simulink model "FW_Matlab_main"  (R2024b)
settings: Solver=ode4  StartTime=0.0  StopTime=inf  FixedStep=0.001  RelTol=1e-3
model workspace (MAT data in the model file):
  freq = 1
libraries: eeGeneralControl x8, slrealtimeiplib x5, cstblocks x3, simulink_extras x2, vrlib x1, aerolibanimutils x1, dspnetwork x1
(part 1 of 2)
settings Model: Creator=s336079  LastModifiedBy=user
settings SolverCC: AlgebraicLoopSolver=TrustRegion
settings DebuggingCC: UnconnectedInputMsg=warning  UnconnectedOutputMsg=warning  UnconnectedLineMsg=warning
settings ModelReferenceCC: EnableRefExpFcnMdlSchedulingChecks=on
settings RTWCC: GPUComputeCapability=3.5

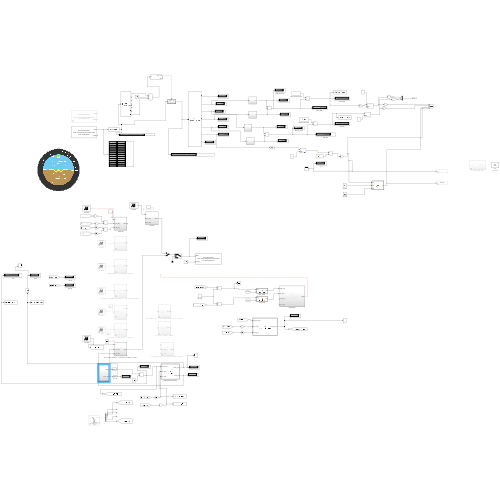
[thumbnail: Simulink's stored preview of the top-level diagram]
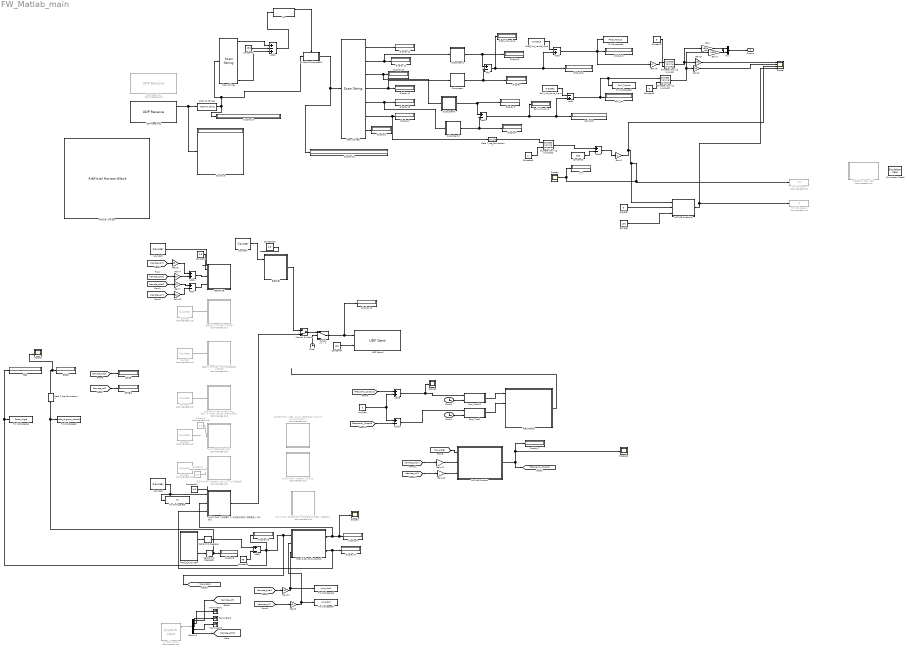
== system FW_Matlab_main ==
  10.27 想做对称推力测试 : Subsystem  Commented=on
  ASCII to String2 : ASCIIToString
  Add{,2,5,7..8,10} (6 alike) : Sum  Inputs=+-
  Add1 : Sum  Inputs=+-+
  Add3 : Sum  Inputs=-+
  Add4 : Sum  Inputs=-+
  Add6 : Sum
  Add9 : Sum
  Artificial Horizon : ArtificialHorizonBlock
  Clock : Clock
  Clock1 : Clock
  Clock2 : Clock
  Constant : Constant  Value=0.8
  Constant1 : Constant  Value=130
  Constant10 : Constant  Value=0.8
  Constant11 : Constant  Value=0.8
  Constant2 : Constant  Commented=on  Value=0.8
  Constant3 : Constant  Value=433
  Constant4 : Constant  Value=100
  Constant5 : Constant  Value=98
  Constant6 : Constant  Commented=on  Value=0.8
  Constant7 : Constant  Value=5
  Constant8 : Constant  Value=5
  Constant9 : Constant  Value=2
  Counter : eeGeneralControl/Counter  Commented=on  CarrCount=Up  Range=[0 1]  Tper=1/5  Tdelay=0  Ts=0.001
  Counter1 : eeGeneralControl/Counter  Commented=on  CarrCount=Up  Range=[0 1]  Tper=1/5  Tdelay=0  Ts=0.001
  Counter2 : eeGeneralControl/Counter  Commented=on  CarrCount=Up  Range=[0 1]  Tper=1/1  Tdelay=0  Ts=0.001
  Counter3 : eeGeneralControl/Counter  Commented=on  CarrCount=Up  Range=[0 1]  Tper=3  Tdelay=0  Ts=0.001
  Counter4 : eeGeneralControl/Counter  Commented=on  CarrCount=Up  Range=[0 1]  Tper=1/5  Tdelay=0  Ts=0.001
  Counter5 : eeGeneralControl/Counter  CarrCount=Up  Range=[0 1]  Tper=1/1  Tdelay=0  Ts=0.001
  Counter6 : eeGeneralControl/Counter  CarrCount=Up  Range=[0 1]  Tper=1/0.1  Tdelay=0  Ts=0.001
  Counter7 : eeGeneralControl/Counter  CarrCount=Up  Range=[0 1]  Tper=1/3  Tdelay=0  Ts=0.001
  Data Type Conversion1 : DataTypeConversion  OutDataTypeStr=double  SaturateOnIntegerOverflow=off  RndMeth=Floor
  Data Type Conversion4 : DataTypeConversion  OutDataTypeStr=double  SaturateOnIntegerOverflow=off  RndMeth=Floor
  Demux1 : Demux  Outputs=5
  Discrete Varying Lowpass : cstblocks/Linear Parameter Varying/Discrete Varying Lowpass  N=1  w0=0  Ts=0.001
  Discrete Varying Lowpass1 : cstblocks/Linear Parameter Varying/Discrete Varying Lowpass  N=1  w0=0  Ts=0.001
  Discrete Varying Lowpass2 : cstblocks/Linear Parameter Varying/Discrete Varying Lowpass  N=1  w0=0  Ts=0.001
  Display{,1..19} (20 alike) : Display
  FWR_Z_AXIS UDP : Subsystem
  Gain : Gain  Gain=1500
  Gain1 : Gain  Gain=1500
  Gain10 : Gain  Gain=20
  Gain11 : Gain  Gain=40
  Gain12 : Gain  Gain=0.01
  Gain13 : Gain  Gain=0.01
  Gain2 : Gain  Gain=-1
  Gain3 : Gain  Gain=40
  Gain4 : Gain  Gain=50
  Gain5 : Gain  Gain=200
  Gain6 : Gain  Gain=200
  Gain7 : Gain  Gain=50
  Gain8 : Gain  Gain=-1
  Gain9 : Gain  Gain=20
  If Action Subsystem2 : Subsystem  TreatAsAtomicUnit=on
  If2 : If  IfExpression=u1 == 0
  Init_Freq : Constant  Value=5
  Joystick Input1 : vrlib/Joystick Input  Commented=on  joyid=1  adjustports=on  forcefeed=off
  MATLAB Function : MATLAB Function  TreatAsAtomicUnit=on
  MATLAB Function6 : MATLAB Function  TreatAsAtomicUnit=on
  Manual Switch1 : ManualSwitch  CurrentSetting=0
  Msc 期间升力最大FWR模式 Msc 期间工作（拍幅：50/-20 扭转角10/50） : Subsystem  Commented=on
  Mux : Mux  Inputs=2
  Pitch_NM : Display
  Pitch_NM1 : Display
  Pitch_init_valve : Display
  Pitch_init_valve_input : Constant  Value=-0.01018
  Radians to Degrees : simulink_extras/Transformations/Radians to Degrees
  Radians to Degrees1 : simulink_extras/Transformations/Radians to Degrees
  Roll_NM : Display
  Roll_NM1 : Display
  Roll_init_valve : Display
  Roll_init_valve_input : Constant  Value=-0.02692
  Saw_Tooth : MATLAB Function  TreatAsAtomicUnit=on
  Saw_Tooth1 : MATLAB Function  TreatAsAtomicUnit=on
  Scan String3 : ScanString  Format="\"%f\\t%f\\t%f\\t%f\\t%f\\t%f\\t%f\\t\""
  Scan String4 : ScanString  Format="\"%f\\t%f\\t%f\\t%f\\t%f\\t%f\\t%f\\t\""
  Scope : Scope  NumInputPorts=4
  Scope1 : Scope  NumInputPorts=2
  Scope{2..4,10} (4 alike) : Scope
  Simulation Pace1 : aerolibanimutils/Simulation Pace  SimulationPace=1  SleepMode=Auto  OutputPaceError=off  SampleTime=0.001
  Subsystem : Subsystem
  Subsystem1 : Subsystem
  Subsystem2 : Subsystem
  Subsystem3 : Subsystem
  Switch : Switch  Criteria=u2 > Threshold  Threshold=5  SaturateOnIntegerOverflow=off  InputSameDT=off
  Terminator1 : Terminator
  Terminator2 : Terminator
  Terminator3 : Terminator
  To Workspace : ToWorkspace  Commented=on  VariableName=Lift  SaveFormat=Timeseries  SampleTime=-1
  To Workspace1 : ToWorkspace  Commented=on  VariableName=Cl  SaveFormat=Timeseries  SampleTime=-1
  To Workspace2 : ToWorkspace  VariableName=Rotor_Angle  SaveFormat=Timeseries  SampleTime=-1
  To Workspace3 : ToWorkspace  VariableName=Rotor_Angular_Velocity  SaveFormat=Timeseries  SampleTime=-1
  To Workspace4 : ToWorkspace  VariableName=Pitch_Torque  SaveFormat=Timeseries  SampleTime=-1
  To Workspace5 : ToWorkspace  VariableName=Roll_Torque  SaveFormat=Timeseries  SampleTime=-1
  To Workspace6 : ToWorkspace  VariableName=Amp_Pitch  SaveFormat=Timeseries  SampleTime=-1
  To Workspace7 : ToWorkspace  VariableName=Amp_Roll  SaveFormat=Timeseries  SampleTime=-1
  To Workspace8 : ToWorkspace  VariableName=Hz  SaveFormat=Timeseries  SampleTime=-1
  Total Pitch Cyclic Control : MATLAB Function  TreatAsAtomicUnit=on
  UDP Receive1 : slrealtimeiplib/UDP Receive  Commented=on  useHostTargetConn=on  ipAddress=10.10.10.15  localPort=2315  rcvWidth=1024  rcvFmAny=off  fmAddress=192.168.0.30  sampleTime=-1  enableMessage=off  maxPackets=1
  UDP Receive2 : slrealtimeiplib/UDP Receive  useHostTargetConn=on  ipAddress=10.10.10.15  localPort=2318  rcvWidth=1024  rcvFmAny=on  fmAddress=192.168.0.51  sampleTime=-1  enableMessage=off  maxPackets=1
  UDP Send1 : slrealtimeiplib/UDP Send  useHostTargetConn=on  toAddress=192.168.0.52  toPort=2316  sampleTime=-1  enableMessage=off  localPort=25001
  两翼分频控制 : Subsystem
  优化中 FWR- 尝试姿态控制-小拍动幅度-新小幅度（周期变距） : Subsystem  Commented=on
  优化中 FWR（当前最优）- 尝试姿态控制（周期变距）124 测王 : Subsystem
  优化中 FWR（当前最优）10.29前 : Subsystem  Commented=on
  优化中 FWR（当前最优）10.29后，改了扭转角度 : Subsystem  Commented=on
  升力 : Display
  "启动测力台 UDP  接收 " : Subsystem  Commented=on
  拍动频率 : Constant  Value=5
  推杆量 : Display
  推杆量1 : Display
  普通扑翼 : Subsystem
  最大拍幅 : Constant  Value=120
  蜻蜓扑动-FWR模式-角度与普通蜻蜓同  45度范围 : Subsystem  Commented=on
  蜻蜓扑动-VTOL模式 45度范围 : Subsystem  Commented=on
  蜻蜓改扑翼 : Subsystem
  角度 : Display
  角速度 : Display
  论文模式 FWR（拍幅：10/-10 扭转角5/25）Cl5.11? 升力没论文说的大 1 : Subsystem  Commented=on
  Output : Outport
  wires:
  Scan String4/1 -> Add1/1
  Scan String3/5 -> Subsystem2/1(In1), Display15/1
  Scan String3/1 -> Display11/1
  Scan String4/7 -> Add1/3
  If2/1 -> If Action Subsystem2/Action
  Scan String3/2 -> Subsystem1/1(In1), Display12/1
  Constant1/1 -> Add1/2
  ASCII to String2/1 -> If Action Subsystem2/1(In1), Scan String4/1, Display10/1
  Add1/1 -> If2/1
  Scan String3/4 -> Subsystem/1(In1), Display14/1
  UDP Receive2/1 -> Display6/1, ASCII to String2/1
  If Action Subsystem2/1(Out1) -> Display16/1, Scan String3/1
  Scan String3/6 -> Data Type Conversion1/1, Display2/1
  Scan String3/3 -> Subsystem3/1(In1), Display13/1
  Scan String3/7 -> Display1/1
  Subsystem/1(Out1) -> Add/2, Display/1
  Subsystem1/1(Out1) -> Add/1, Display3/1
  Add/1 -> Add3/2, Pitch_NM1/1, Pitch_init_valve/1
  Subsystem3/1(Out1) -> Display5/1, Add2/1
  Subsystem2/1(Out1) -> Add2/2, Display4/1
  Pitch_init_valve_input/1 -> Add3/1
  Add3/1 -> To Workspace4/1, Gain8/1, Pitch_NM/1
  Roll_init_valve_input/1 -> Add4/1
  Add4/1 -> To Workspace5/1, Discrete Varying Lowpass1/1, Roll_NM/1
  Add2/1 -> Roll_init_valve/1, Add4/2, Roll_NM1/1
  Mux/1 -> Output/1
  Gain/1 -> Mux/2
  Gain1/1 -> Mux/1
  Constant3/1 -> Add5/2
  Add5/1 -> Gain2/1
  Gain5/1 -> Scope/1
  Gain6/1 -> Scope/2
  Demux1/3 -> Terminator2/1
  Demux1/2 -> Terminator1/1
  Demux1/4 -> Terminator3/1
  Demux1/5 -> [remote_pitch]
  Demux1/1 -> [remote_roll]
  Joystick Input1/1 -> Demux1/1
  拍动频率/1 -> MATLAB Function6/2(freq)
  最大拍幅/1 -> MATLAB Function6/3(Amp)
  MATLAB Function6/1(Cl) -> Scope/4, To Workspace1/1
  Counter/1 -> 蜻蜓扑动-VTOL模式 45度范围/1(In1)
  Counter1/1 -> 蜻蜓扑动-FWR模式-角度与普通蜻蜓同  45度范围/1(In1)
  Constant4/1 -> UDP Send1/2
  Switch/1 -> Display19/1, UDP Send1/1
  Counter2/1 -> Msc 期间升力最大FWR模式 Msc 期间工作（拍幅：50/-20 扭转角10/50）/1(In1)
  Clock/1 -> Switch/2
  Manual Switch1/1 -> Switch/1
  Counter3/1 -> ?
  优化中 FWR（当前最优）- 尝试姿态控制（周期变距）124 测王/1(Signal) -> Manual Switch1/2
  Counter4/1 -> 优化中 FWR（当前最优）10.29后，改了扭转角度/1(In1)
  Counter5/1 -> ?
  普通扑翼/1(Signal) -> Manual Switch1/1
  FWR_Z_AXIS UDP/1(Angle) -> Radians to Degrees/1
  Counter6/1 -> 优化中 FWR（当前最优）- 尝试姿态控制（周期变距）124 测王/1(In1), To Workspace8/1
  Total Pitch Cyclic Control/1(blade_right) -> 优化中 FWR（当前最优）- 尝试姿态控制（周期变距）124 测王/2(R_Pit_Ang), Scope2/1, Display9/1
  Total Pitch Cyclic Control/2(blade_left) -> 优化中 FWR（当前最优）- 尝试姿态控制（周期变距）124 测王/3(L_Pit_Ang), Display17/1
  Constant2/1 -> ?
  Data Type Conversion4/1 -> Scope1/2, 角速度/1
  [remote_pitch] -> Gain4/1
  Gain4/1 -> Add6/2
  [remote_pitch] -> Gain7/1
  Gain7/1 -> Add7/1
  Constant/1 -> 蜻蜓改扑翼/1(In1)
  Gain8/1 -> Discrete Varying Lowpass/1
  Add6/1 -> 蜻蜓改扑翼/2(R_Pit_Ang)
  [remote_roll] -> Gain9/1
  [remote_roll] -> Gain10/1
  Add7/1 -> 蜻蜓改扑翼/3(L_Pit_Ang)
  Gain9/1 -> Add6/1
  Gain10/1 -> Add7/2
  FWR_Z_AXIS UDP/2(Angle_Vel) -> Radians to Degrees1/1
  Radians to Degrees/1 -> Add8/1
  Radians to Degrees1/1 -> To Workspace3/1, Data Type Conversion4/1, Display8/1
  Constant5/1 -> Add8/2
  [remote_pitch] -> Gain11/1
  Gain3/1 -> To Workspace7/1, Total Pitch Cyclic Control/2(Amp_Roll)
  [remote_pitch] -> 推杆量/1
  [remote_roll] -> Gain3/1
  Discrete Varying Lowpass/1 -> Gain/1, Gain5/1
  Discrete Varying Lowpass1/1 -> Gain1/1, Gain6/1
  Constant7/1 -> Discrete Varying Lowpass/2
  Constant8/1 -> Discrete Varying Lowpass1/2
  Gain11/1 -> To Workspace6/1, Total Pitch Cyclic Control/3(Amp_Pitch)
  [remote_roll] -> 推杆量1/1
  Discrete Varying Lowpass2/1 -> Add5/1
  Constant9/1 -> Discrete Varying Lowpass2/2
  Data Type Conversion1/1 -> Discrete Varying Lowpass2/1
  Counter7/1 -> 普通扑翼/1(In1)
  两翼分频控制/1(Signal) -> ?
  [Az_Angle] -> MATLAB Function/1(Azimuth_Angle)
  MATLAB Function/1(Freq_diff_out) -> [Frequency_Output], Scope10/1, Display7/1
  Clock1/1 -> Saw_Tooth/2(t)
  Add10/1 -> Saw_Tooth/1(freq)
  Saw_Tooth/1(Out) -> 两翼分频控制/2(Left_Freq)
  Clock2/1 -> Saw_Tooth1/2(t)
  Saw_Tooth1/1(Out) -> 两翼分频控制/1(Right_Freq)
  Add9/1 -> Scope3/1, Saw_Tooth1/1(freq)
  [Frequency_Output] -> Add10/2
  Init_Freq/1 -> Add9/2, Add10/1
  [Frequency_Output] -> Add9/1
  [remote_pitch] -> Gain12/1
  [remote_roll] -> Gain13/1
  Gain12/1 -> MATLAB Function/2(force_req_x)
  Gain13/1 -> MATLAB Function/3(force_req_y)
  Add8/1 -> To Workspace2/1, 角度/1, Display18/1, [Az_Angle], Total Pitch Cyclic Control/1(azimuth_ang)
  Gain2/1 -> MATLAB Function6/1(Lift), To Workspace/1, Scope4/1, 升力/1, Scope/3
  Constant6/1 -> 10.27 想做对称推力测试/1(In1)
  Constant10/1 -> ?
  Constant11/1 -> ?

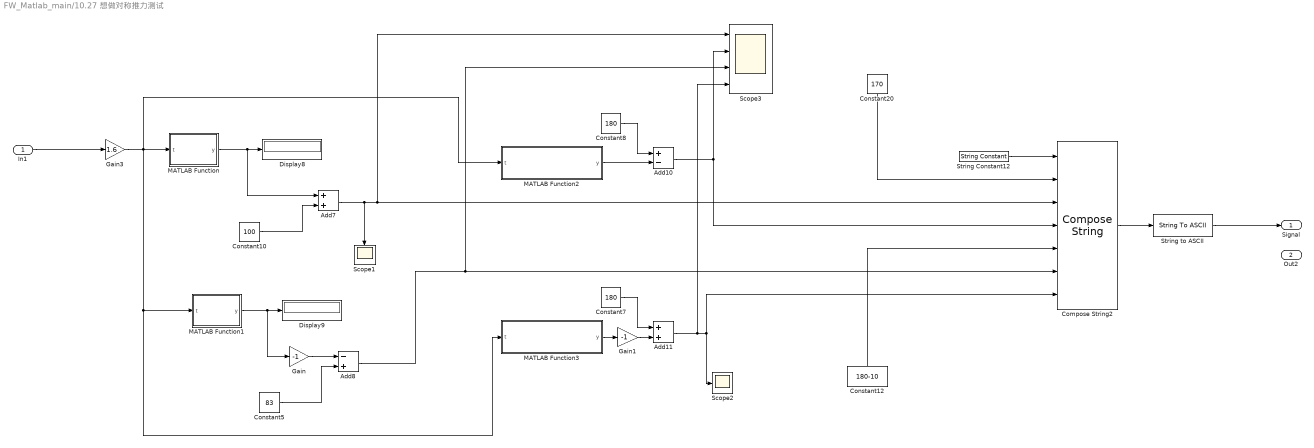
== system FW_Matlab_main/10.27 想做对称推力测试 ==
  In1 : Inport
  Add10 : Sum  Inputs=+-
  Add11 : Sum
  Add7 : Sum
  Add8 : Sum  Inputs=-+
  Compose String2 : ComposeString  Format="\"%s%f %f %f %f %f %f\""
  Constant10 : Constant  Value=100
  Constant12 : Constant  Value=180-10
  Constant20 : Constant  Value=170
  Constant5 : Constant  Value=83
  Constant7 : Constant  Value=180
  Constant8 : Constant  Value=180
  Display8 : Display
  Display9 : Display
  Gain : Gain  Gain=-1
  Gain1 : Gain  Gain=-1
  Gain3 : Gain  Gain=1.6
  MATLAB Function : MATLAB Function  TreatAsAtomicUnit=on
  MATLAB Function1 : MATLAB Function  TreatAsAtomicUnit=on
  MATLAB Function2 : MATLAB Function  TreatAsAtomicUnit=on
  MATLAB Function3 : MATLAB Function  TreatAsAtomicUnit=on
  Scope1 : Scope
  Scope2 : Scope
  Scope3 : Scope  NumInputPorts=4
  String Constant12 : StringConstant  String="\"T\""
  String to ASCII : StringToASCII  OutputVectorSize=80
  Signal : Outport
  Out2 : Outport  Port=2
  wires:
  Gain3/1 -> MATLAB Function3/1(t), MATLAB Function1/1(t), MATLAB Function2/1(t), MATLAB Function/1(t)
  String Constant12/1 -> Compose String2/1
  MATLAB Function/1(y) -> Add7/1, Display8/1
  Constant20/1 -> Compose String2/2
  MATLAB Function2/1(y) -> Add10/2
  Constant10/1 -> Add7/2
  Constant8/1 -> Add10/1
  MATLAB Function3/1(y) -> Gain1/1
  MATLAB Function1/1(y) -> Gain/1, Display9/1
  String to ASCII/1 -> Signal/1
  Compose String2/1 -> String to ASCII/1
  Constant5/1 -> Add8/2
  Constant7/1 -> Add11/1
  Constant12/1 -> Compose String2/5
  In1/1 -> Gain3/1
  Gain/1 -> Add8/1
  Gain1/1 -> Add11/2
  Add7/1 -> Scope1/1, Compose String2/3, Scope3/1
  Add8/1 -> Compose String2/6, Scope3/3
  Add10/1 -> Compose String2/4, Scope3/2
  Add11/1 -> Compose String2/7, Scope2/1, Scope3/4

== system FW_Matlab_main/FWR_Z_AXIS UDP ==
  ASCII to String1 : ASCIIToString
  Add7 : Sum  Inputs=+-+
  Constant2 : Constant  Value=130
  If Action Subsystem1 : Subsystem  TreatAsAtomicUnit=on
  If1 : If  IfExpression=u1 == 0
  Scan String1 : ScanString  Format="\"%f\\t%f\\t%f\\t%f\\t\""
  Scan String2 : ScanString  Format="\"%f\\t%f\\t%f\\t%f\\t\""
  UDP Receive1 : slrealtimeiplib/UDP Receive  useHostTargetConn=on  ipAddress=10.10.10.15  localPort=2316  rcvWidth=1024  rcvFmAny=on  fmAddress=192.168.0.52  sampleTime=-1  enableMessage=off  maxPackets=1
  UDP Receive2 : slrealtimeiplib/UDP Receive  Commented=on  useHostTargetConn=on  ipAddress=10.10.10.15  localPort=2316  rcvWidth=1024  rcvFmAny=off  fmAddress=192.168.0.31  sampleTime=-1  enableMessage=off  maxPackets=1
  Angle : Outport
  Angle_Vel : Outport  Port=2
  wires:
  Scan String1/1 -> Add7/1
  ASCII to String1/1 -> If Action Subsystem1/1(In1), Scan String1/1
  UDP Receive1/1 -> ASCII to String1/1
  Scan String1/4 -> Add7/3
  If Action Subsystem1/1(Out1) -> Scan String2/1
  Add7/1 -> If1/1
  Scan String2/3 -> Angle_Vel/1
  Constant2/1 -> Add7/2
  If1/1 -> If Action Subsystem1/Action
  Scan String2/2 -> Angle/1

== system FW_Matlab_main/If Action Subsystem2 ==
  In1 : Inport
  Action Port : ActionPort  ActionPortLabel=if(u1 == 0)
  Out1 : Outport
  wires:
  In1/1 -> Out1/1

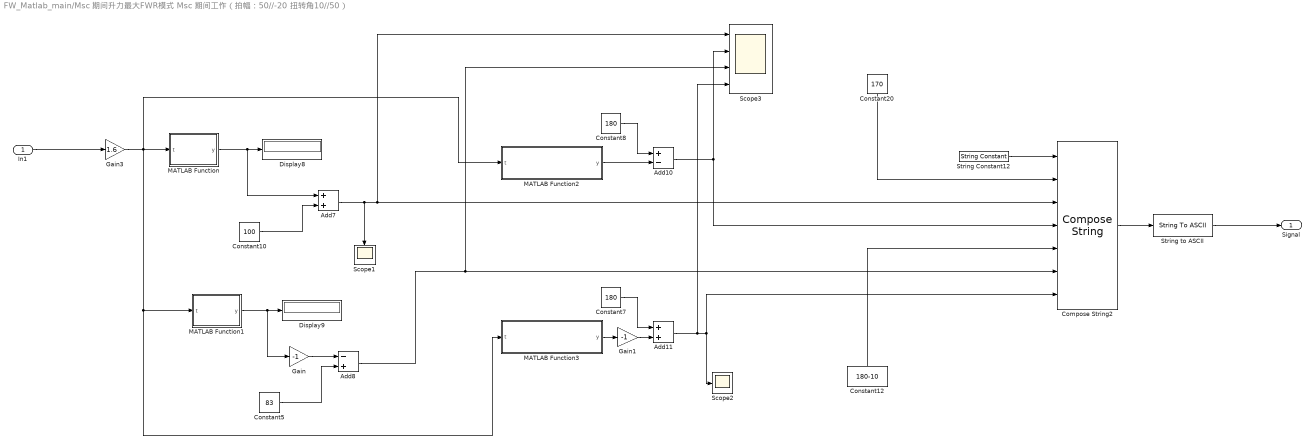
== system FW_Matlab_main/Msc 期间升力最大FWR模式 Msc 期间工作（拍幅：50//-20 扭转角10//50） ==
  In1 : Inport
  Add10 : Sum  Inputs=+-
  Add11 : Sum
  Add7 : Sum
  Add8 : Sum  Inputs=-+
  Compose String2 : ComposeString  Format="\"%s%f %f %f %f %f %f\""
  Constant10 : Constant  Value=100
  Constant12 : Constant  Value=180-10
  Constant20 : Constant  Value=170
  Constant5 : Constant  Value=83
  Constant7 : Constant  Value=180
  Constant8 : Constant  Value=180
  Display8 : Display
  Display9 : Display
  Gain : Gain  Gain=-1
  Gain1 : Gain  Gain=-1
  Gain3 : Gain  Gain=1.6
  MATLAB Function : MATLAB Function  TreatAsAtomicUnit=on
  MATLAB Function1 : MATLAB Function  TreatAsAtomicUnit=on
  MATLAB Function2 : MATLAB Function  TreatAsAtomicUnit=on
  MATLAB Function3 : MATLAB Function  TreatAsAtomicUnit=on
  Scope1 : Scope
  Scope2 : Scope
  Scope3 : Scope  NumInputPorts=4
  String Constant12 : StringConstant  String="\"T\""
  String to ASCII : StringToASCII  OutputVectorSize=80
  Signal : Outport
  wires:
  Gain3/1 -> MATLAB Function3/1(t), MATLAB Function1/1(t), MATLAB Function2/1(t), MATLAB Function/1(t)
  String Constant12/1 -> Compose String2/1
  MATLAB Function/1(y) -> Add7/1, Display8/1
  Constant20/1 -> Compose String2/2
  MATLAB Function2/1(y) -> Add10/2
  Constant10/1 -> Add7/2
  Constant8/1 -> Add10/1
  MATLAB Function3/1(y) -> Gain1/1
  MATLAB Function1/1(y) -> Gain/1, Display9/1
  String to ASCII/1 -> Signal/1
  Compose String2/1 -> String to ASCII/1
  Constant5/1 -> Add8/2
  Constant7/1 -> Add11/1
  Constant12/1 -> Compose String2/5
  In1/1 -> Gain3/1
  Gain/1 -> Add8/1
  Gain1/1 -> Add11/2
  Add7/1 -> Scope1/1, Compose String2/3, Scope3/1
  Add8/1 -> Compose String2/6, Scope3/3
  Add10/1 -> Compose String2/4, Scope3/2
  Add11/1 -> Compose String2/7, Scope2/1, Scope3/4

== system FW_Matlab_main/Subsystem ==
  In1 : Inport
  Gain : Gain  Gain=(1/1000)*9.81
  Gain1 : Gain  Gain=45*(1/1000)
  Out1 : Outport
  wires:
  Gain/1 -> Gain1/1
  In1/1 -> Gain/1
  Gain1/1 -> Out1/1

== system FW_Matlab_main/Subsystem1 ==
  In1 : Inport
  Gain : Gain  Gain=(1/1000)*9.81
  Gain1 : Gain  Gain=45*(1/1000)
  Out1 : Outport
  wires:
  Gain/1 -> Gain1/1
  In1/1 -> Gain/1
  Gain1/1 -> Out1/1

== system FW_Matlab_main/Subsystem2 ==
  In1 : Inport
  Gain : Gain  Gain=(1/1000)*9.81
  Gain1 : Gain  Gain=45*(1/1000)
  Out1 : Outport
  wires:
  Gain/1 -> Gain1/1
  In1/1 -> Gain/1
  Gain1/1 -> Out1/1

== system FW_Matlab_main/Subsystem3 ==
  In1 : Inport
  Gain : Gain  Gain=(1/1000)*9.81
  Gain1 : Gain  Gain=45*(1/1000)
  Out1 : Outport
  wires:
  Gain/1 -> Gain1/1
  In1/1 -> Gain/1
  Gain1/1 -> Out1/1

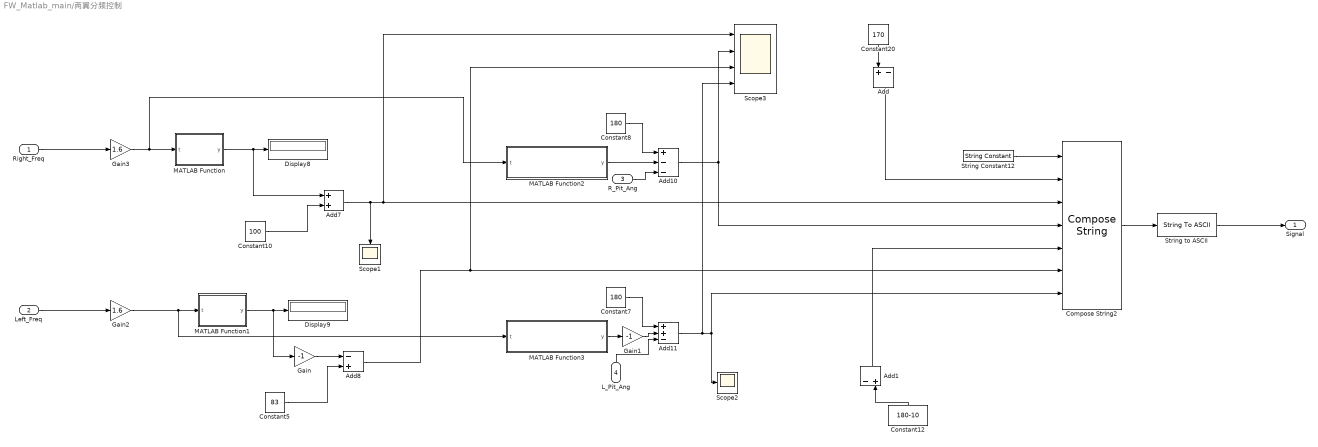
== system FW_Matlab_main/两翼分频控制 ==
  Right_Freq : Inport
  Left_Freq : Inport  Port=2
  R_Pit_Ang : Inport  Port=3
  L_Pit_Ang : Inport  Port=4
  Add : Sum  Inputs=+-
  Add1 : Sum  Inputs=-+
  Add10 : Sum  Inputs=+--
  Add11 : Sum  Inputs=++-
  Add7 : Sum
  Add8 : Sum  Inputs=-+
  Compose String2 : ComposeString  Format="\"%s%f %f %f %f %f %f\""
  Constant10 : Constant  Value=100
  Constant12 : Constant  Value=180-10
  Constant20 : Constant  Value=170
  Constant5 : Constant  Value=83
  Constant7 : Constant  Value=180
  Constant8 : Constant  Value=180
  Display8 : Display
  Display9 : Display
  Gain : Gain  Gain=-1
  Gain1 : Gain  Gain=-1
  Gain2 : Gain  Gain=1.6
  Gain3 : Gain  Gain=1.6
  MATLAB Function : MATLAB Function  TreatAsAtomicUnit=on
  MATLAB Function1 : MATLAB Function  TreatAsAtomicUnit=on
  MATLAB Function2 : MATLAB Function  TreatAsAtomicUnit=on
  MATLAB Function3 : MATLAB Function  TreatAsAtomicUnit=on
  Scope1 : Scope
  Scope2 : Scope
  Scope3 : Scope  NumInputPorts=4
  String Constant12 : StringConstant  String="\"T\""
  String to ASCII : StringToASCII  OutputVectorSize=80
  Signal : Outport
  wires:
  Gain3/1 -> MATLAB Function2/1(t), MATLAB Function/1(t)
  String Constant12/1 -> Compose String2/1
  MATLAB Function/1(y) -> Add7/1, Display8/1
  Add/1 -> Compose String2/2
  MATLAB Function2/1(y) -> Add10/2
  Constant10/1 -> Add7/2
  Constant8/1 -> Add10/1
  MATLAB Function3/1(y) -> Gain1/1
  MATLAB Function1/1(y) -> Gain/1, Display9/1
  String to ASCII/1 -> Signal/1
  Compose String2/1 -> String to ASCII/1
  Constant5/1 -> Add8/2
  Constant7/1 -> Add11/1
  Add1/1 -> Compose String2/5
  Right_Freq/1 -> Gain3/1
  Gain/1 -> Add8/1
  Gain1/1 -> Add11/2
  Add7/1 -> Scope1/1, Compose String2/3, Scope3/1
  Add8/1 -> Compose String2/6, Scope3/3
  Add10/1 -> Scope3/2, Compose String2/4
  Add11/1 -> Compose String2/7, Scope2/1, Scope3/4
  Constant20/1 -> Add/1
  Constant12/1 -> Add1/2
  R_Pit_Ang/1 -> Add10/3
  L_Pit_Ang/1 -> Add11/3
  Left_Freq/1 -> Gain2/1
  Gain2/1 -> MATLAB Function3/1(t), MATLAB Function1/1(t)

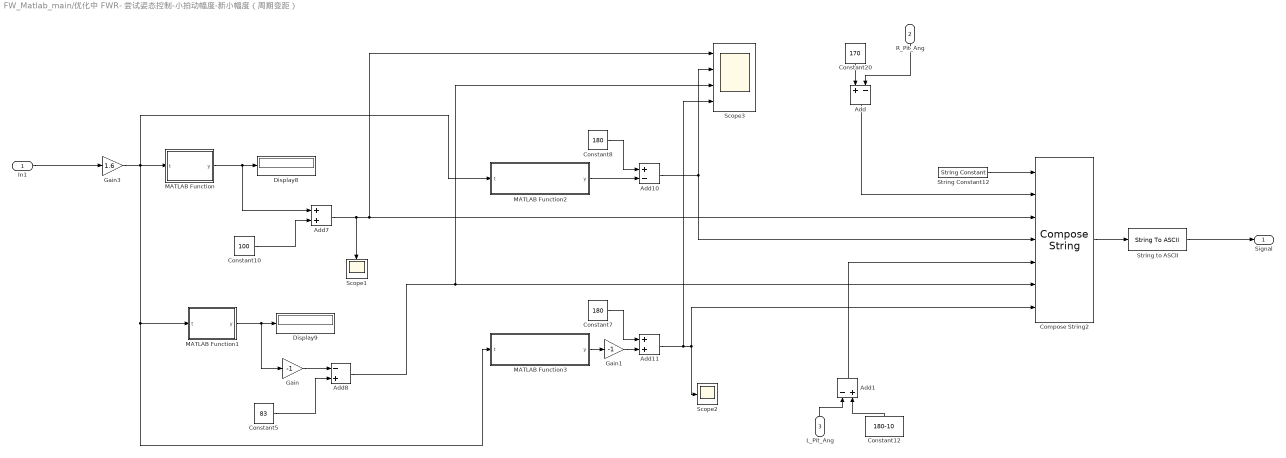
== system FW_Matlab_main/优化中 FWR- 尝试姿态控制-小拍动幅度-新小幅度（周期变距） ==
  In1 : Inport
  R_Pit_Ang : Inport  Port=2
  L_Pit_Ang : Inport  Port=3
  Add : Sum  Inputs=+-
  Add1 : Sum  Inputs=-+
  Add10 : Sum  Inputs=+-
  Add11 : Sum
  Add7 : Sum
  Add8 : Sum  Inputs=-+
  Compose String2 : ComposeString  Format="\"%s%f %f %f %f %f %f\""
  Constant10 : Constant  Value=100
  Constant12 : Constant  Value=180-10
  Constant20 : Constant  Value=170
  Constant5 : Constant  Value=83
  Constant7 : Constant  Value=180
  Constant8 : Constant  Value=180
  Display8 : Display
  Display9 : Display
  Gain : Gain  Gain=-1
  Gain1 : Gain  Gain=-1
  Gain3 : Gain  Gain=1.6
  MATLAB Function : MATLAB Function  TreatAsAtomicUnit=on
  MATLAB Function1 : MATLAB Function  TreatAsAtomicUnit=on
  MATLAB Function2 : MATLAB Function  TreatAsAtomicUnit=on
  MATLAB Function3 : MATLAB Function  TreatAsAtomicUnit=on
  Scope1 : Scope
  Scope2 : Scope
  Scope3 : Scope  NumInputPorts=4
  String Constant12 : StringConstant  String="\"T\""
  String to ASCII : StringToASCII  OutputVectorSize=80
  Signal : Outport
  wires:
  Gain3/1 -> MATLAB Function3/1(t), MATLAB Function1/1(t), MATLAB Function2/1(t), MATLAB Function/1(t)
  String Constant12/1 -> Compose String2/1
  MATLAB Function/1(y) -> Add7/1, Display8/1
  Add/1 -> Compose String2/2
  MATLAB Function2/1(y) -> Add10/2
  Constant10/1 -> Add7/2
  Constant8/1 -> Add10/1
  MATLAB Function3/1(y) -> Gain1/1
  MATLAB Function1/1(y) -> Gain/1, Display9/1
  String to ASCII/1 -> Signal/1
  Compose String2/1 -> String to ASCII/1
  Constant5/1 -> Add8/2
  Constant7/1 -> Add11/1
  Add1/1 -> Compose String2/5
  In1/1 -> Gain3/1
  Gain/1 -> Add8/1
  Gain1/1 -> Add11/2
  Add7/1 -> Scope1/1, Compose String2/3, Scope3/1
  Add8/1 -> Compose String2/6, Scope3/3
  Add10/1 -> Compose String2/4, Scope3/2
  Add11/1 -> Compose String2/7, Scope2/1, Scope3/4
  Constant20/1 -> Add/1
  R_Pit_Ang/1 -> Add/2
  Constant12/1 -> Add1/2
  L_Pit_Ang/1 -> Add1/1

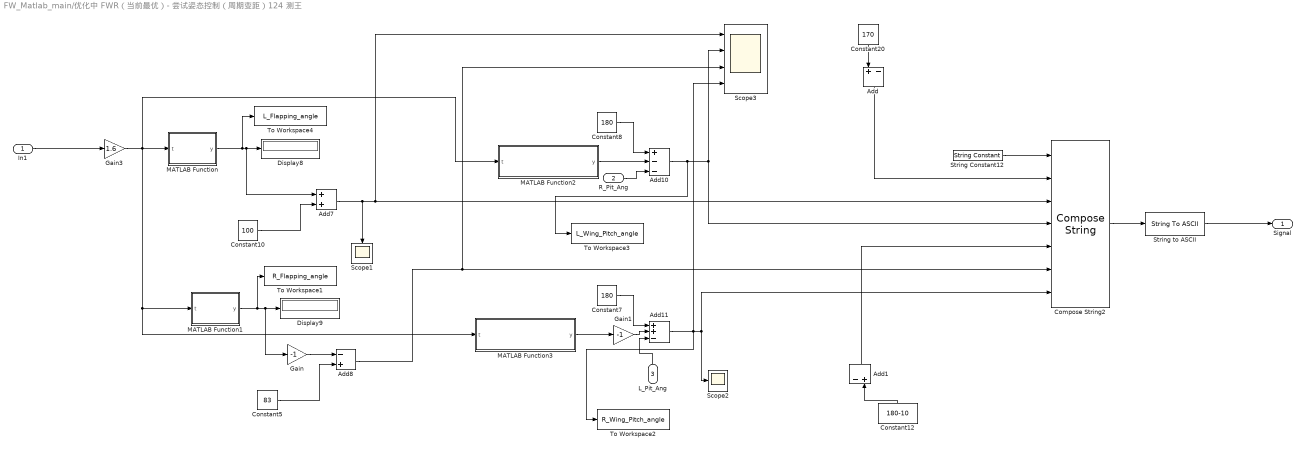
== system FW_Matlab_main/优化中 FWR（当前最优）- 尝试姿态控制（周期变距）124 测王 ==
  In1 : Inport
  R_Pit_Ang : Inport  Port=2
  L_Pit_Ang : Inport  Port=3
  Add : Sum  Inputs=+-
  Add1 : Sum  Inputs=-+
  Add10 : Sum  Inputs=+--
  Add11 : Sum  Inputs=++-
  Add7 : Sum
  Add8 : Sum  Inputs=-+
  Compose String2 : ComposeString  Format="\"%s%f %f %f %f %f %f\""
  Constant10 : Constant  Value=100
  Constant12 : Constant  Value=180-10
  Constant20 : Constant  Value=170
  Constant5 : Constant  Value=83
  Constant7 : Constant  Value=180
  Constant8 : Constant  Value=180
  Display8 : Display
  Display9 : Display
  Gain : Gain  Gain=-1
  Gain1 : Gain  Gain=-1
  Gain3 : Gain  Gain=1.6
  MATLAB Function : MATLAB Function  TreatAsAtomicUnit=on
  MATLAB Function1 : MATLAB Function  TreatAsAtomicUnit=on
  MATLAB Function2 : MATLAB Function  TreatAsAtomicUnit=on
  MATLAB Function3 : MATLAB Function  TreatAsAtomicUnit=on
  Scope1 : Scope
  Scope2 : Scope
  Scope3 : Scope  NumInputPorts=4
  String Constant12 : StringConstant  String="\"T\""
  String to ASCII : StringToASCII  OutputVectorSize=80
  To Workspace1 : ToWorkspace  VariableName=R_Flapping_angle  SaveFormat=Timeseries  SampleTime=-1
  To Workspace2 : ToWorkspace  VariableName=R_Wing_Pitch_angle  SaveFormat=Timeseries  SampleTime=-1
  To Workspace3 : ToWorkspace  VariableName=L_Wing_Pitch_angle  SaveFormat=Timeseries  SampleTime=-1
  To Workspace4 : ToWorkspace  VariableName=L_Flapping_angle  SaveFormat=Timeseries  SampleTime=-1
  Signal : Outport
  wires:
  Gain3/1 -> MATLAB Function3/1(t), MATLAB Function1/1(t), MATLAB Function2/1(t), MATLAB Function/1(t)
  String Constant12/1 -> Compose String2/1
  MATLAB Function/1(y) -> To Workspace4/1, Add7/1, Display8/1
  Add/1 -> Compose String2/2
  MATLAB Function2/1(y) -> Add10/2
  Constant10/1 -> Add7/2
  Constant8/1 -> Add10/1
  MATLAB Function1/1(y) -> To Workspace1/1, Gain/1, Display9/1
  String to ASCII/1 -> Signal/1
  Compose String2/1 -> String to ASCII/1
  Constant5/1 -> Add8/2
  Constant7/1 -> Add11/1
  Add1/1 -> Compose String2/5
  In1/1 -> Gain3/1
  Gain/1 -> Add8/1
  Gain1/1 -> Add11/2
  Add7/1 -> Scope1/1, Compose String2/3, Scope3/1
  Add8/1 -> Compose String2/6, Scope3/3
  Add10/1 -> To Workspace3/1, Scope3/2, Compose String2/4
  Add11/1 -> To Workspace2/1, Compose String2/7, Scope2/1, Scope3/4
  Constant20/1 -> Add/1
  Constant12/1 -> Add1/2
  R_Pit_Ang/1 -> Add10/3
  L_Pit_Ang/1 -> Add11/3
  MATLAB Function3/1(y) -> Gain1/1

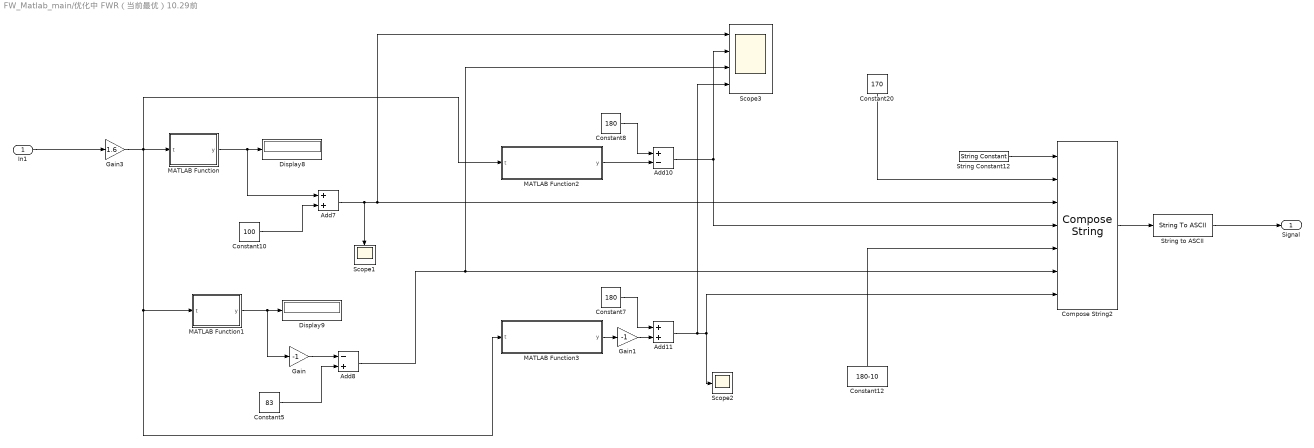
== system FW_Matlab_main/优化中 FWR（当前最优）10.29前 ==
  In1 : Inport
  Add10 : Sum  Inputs=+-
  Add11 : Sum
  Add7 : Sum
  Add8 : Sum  Inputs=-+
  Compose String2 : ComposeString  Format="\"%s%f %f %f %f %f %f\""
  Constant10 : Constant  Value=100
  Constant12 : Constant  Value=180-10
  Constant20 : Constant  Value=170
  Constant5 : Constant  Value=83
  Constant7 : Constant  Value=180
  Constant8 : Constant  Value=180
  Display8 : Display
  Display9 : Display
  Gain : Gain  Gain=-1
  Gain1 : Gain  Gain=-1
  Gain3 : Gain  Gain=1.6
  MATLAB Function : MATLAB Function  TreatAsAtomicUnit=on
  MATLAB Function1 : MATLAB Function  TreatAsAtomicUnit=on
  MATLAB Function2 : MATLAB Function  TreatAsAtomicUnit=on
  MATLAB Function3 : MATLAB Function  TreatAsAtomicUnit=on
  Scope1 : Scope
  Scope2 : Scope
  Scope3 : Scope  NumInputPorts=4
  String Constant12 : StringConstant  String="\"T\""
  String to ASCII : StringToASCII  OutputVectorSize=80
  Signal : Outport
  wires:
  Gain3/1 -> MATLAB Function3/1(t), MATLAB Function1/1(t), MATLAB Function2/1(t), MATLAB Function/1(t)
  String Constant12/1 -> Compose String2/1
  MATLAB Function/1(y) -> Add7/1, Display8/1
  Constant20/1 -> Compose String2/2
  MATLAB Function2/1(y) -> Add10/2
  Constant10/1 -> Add7/2
  Constant8/1 -> Add10/1
  MATLAB Function3/1(y) -> Gain1/1
  MATLAB Function1/1(y) -> Gain/1, Display9/1
  String to ASCII/1 -> Signal/1
  Compose String2/1 -> String to ASCII/1
  Constant5/1 -> Add8/2
  Constant7/1 -> Add11/1
  Constant12/1 -> Compose String2/5
  In1/1 -> Gain3/1
  Gain/1 -> Add8/1
  Gain1/1 -> Add11/2
  Add7/1 -> Scope1/1, Compose String2/3, Scope3/1
  Add8/1 -> Compose String2/6, Scope3/3
  Add10/1 -> Compose String2/4, Scope3/2
  Add11/1 -> Compose String2/7, Scope2/1, Scope3/4

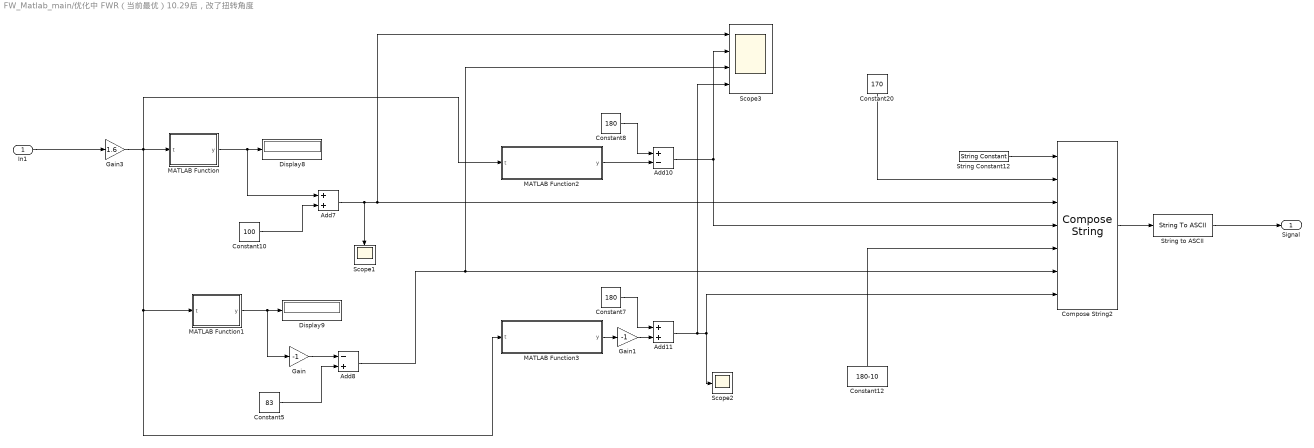
== system FW_Matlab_main/优化中 FWR（当前最优）10.29后，改了扭转角度 ==
  In1 : Inport
  Add10 : Sum  Inputs=+-
  Add11 : Sum
  Add7 : Sum
  Add8 : Sum  Inputs=-+
  Compose String2 : ComposeString  Format="\"%s%f %f %f %f %f %f\""
  Constant10 : Constant  Value=100
  Constant12 : Constant  Value=180-10
  Constant20 : Constant  Value=170
  Constant5 : Constant  Value=83
  Constant7 : Constant  Value=180
  Constant8 : Constant  Value=180
  Display8 : Display
  Display9 : Display
  Gain : Gain  Gain=-1
  Gain1 : Gain  Gain=-1
  Gain3 : Gain  Gain=1.6
  MATLAB Function : MATLAB Function  TreatAsAtomicUnit=on
  MATLAB Function1 : MATLAB Function  TreatAsAtomicUnit=on
  MATLAB Function2 : MATLAB Function  TreatAsAtomicUnit=on
  MATLAB Function3 : MATLAB Function  TreatAsAtomicUnit=on
  Scope1 : Scope
  Scope2 : Scope
  Scope3 : Scope  NumInputPorts=4
  String Constant12 : StringConstant  String="\"T\""
  String to ASCII : StringToASCII  OutputVectorSize=80
  Signal : Outport
  wires:
  Gain3/1 -> MATLAB Function3/1(t), MATLAB Function1/1(t), MATLAB Function2/1(t), MATLAB Function/1(t)
  String Constant12/1 -> Compose String2/1
  MATLAB Function/1(y) -> Add7/1, Display8/1
  Constant20/1 -> Compose String2/2
  MATLAB Function2/1(y) -> Add10/2
  Constant10/1 -> Add7/2
  Constant8/1 -> Add10/1
  MATLAB Function3/1(y) -> Gain1/1
  MATLAB Function1/1(y) -> Gain/1, Display9/1
  String to ASCII/1 -> Signal/1
  Compose String2/1 -> String to ASCII/1
  Constant5/1 -> Add8/2
  Constant7/1 -> Add11/1
  Constant12/1 -> Compose String2/5
  In1/1 -> Gain3/1
  Gain/1 -> Add8/1
  Gain1/1 -> Add11/2
  Add7/1 -> Scope1/1, Compose String2/3, Scope3/1
  Add8/1 -> Compose String2/6, Scope3/3
  Add10/1 -> Compose String2/4, Scope3/2
  Add11/1 -> Compose String2/7, Scope2/1, Scope3/4

== system FW_Matlab_main/启动测力台 UDP  接收  ==
  Clock2 : Clock
  Floor : Rounding
  If Action Subsystem4 : Subsystem  TreatAsAtomicUnit=on
  String Constant6 : StringConstant  String="\"S\""
  String to ASCII9 : StringToASCII
  Switch Case : SwitchCase  CaseConditions={0,1,2}
  UDP Send1 : dspnetwork/UDP Send  remoteURL='192.168.0.144'  remotePort=2315  localURL='0.0.0.0'  localPortSource=Automatically determine  localPort=-1  sampletime=-1  blockPlatform=[]  separateLengthPort=0
      settings: SourceProductName=Simulink
  wires:
  String to ASCII9/1 -> If Action Subsystem4/1(In1)
  Clock2/1 -> Floor/1
  If Action Subsystem4/1(Out1) -> UDP Send1/1
  String Constant6/1 -> String to ASCII9/1
  Floor/1 -> Switch Case/1
  Switch Case/1 -> If Action Subsystem4/Action

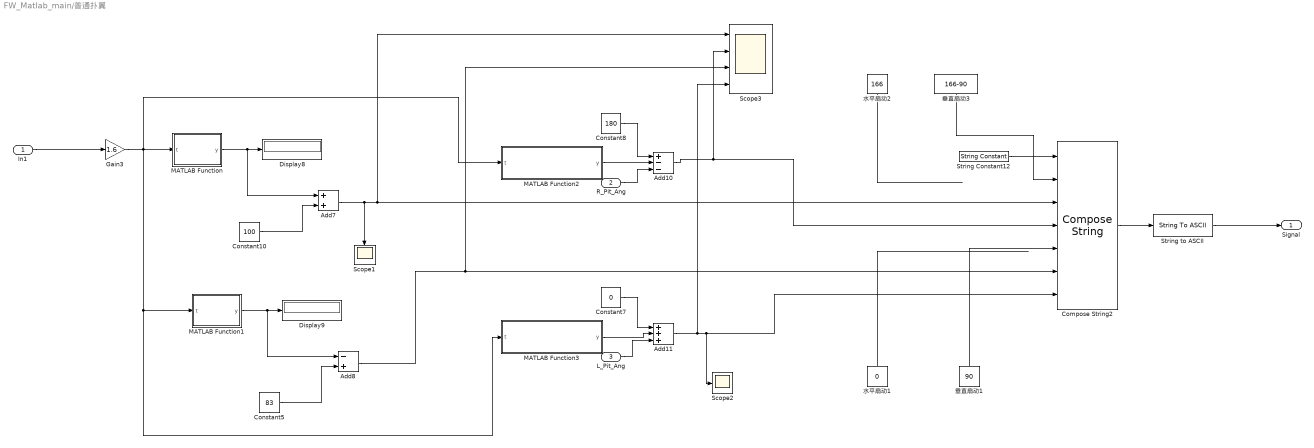
== system FW_Matlab_main/普通扑翼 ==
  In1 : Inport
  R_Pit_Ang : Inport  Port=2
  L_Pit_Ang : Inport  Port=3
  Add10 : Sum  Inputs=+--
  Add11 : Sum  Inputs=+++
  Add7 : Sum
  Add8 : Sum  Inputs=-+
  Compose String2 : ComposeString  Format="\"%s%f %f %f %f %f %f\""
  Constant10 : Constant  Value=100
  Constant5 : Constant  Value=83
  Constant7 : Constant  Value=0
  Constant8 : Constant  Value=180
  Display8 : Display
  Display9 : Display
  Gain3 : Gain  Gain=1.6
  MATLAB Function : MATLAB Function  TreatAsAtomicUnit=on
  MATLAB Function1 : MATLAB Function  TreatAsAtomicUnit=on
  MATLAB Function2 : MATLAB Function  TreatAsAtomicUnit=on
  MATLAB Function3 : MATLAB Function  TreatAsAtomicUnit=on
  Scope1 : Scope
  Scope2 : Scope
  Scope3 : Scope  NumInputPorts=4
  String Constant12 : StringConstant  String="\"T\""
  String to ASCII : StringToASCII  OutputVectorSize=80
  垂直扇动1 : Constant  Value=90
  垂直扇动3 : Constant  Value=166-90
  水平扇动1 : Constant  Value=0
  水平扇动2 : Constant  Value=166
  Signal : Outport
  wires:
  Add11/1 -> Compose String2/7, Scope2/1, Scope3/4
  Gain3/1 -> MATLAB Function3/1(t), MATLAB Function1/1(t), MATLAB Function2/1(t), MATLAB Function/1(t)
  String Constant12/1 -> Compose String2/1
  Add7/1 -> Scope1/1, Compose String2/3, Scope3/1
  MATLAB Function/1(y) -> Add7/1, Display8/1
  水平扇动2/1 -> ?
  MATLAB Function2/1(y) -> Add10/2
  Constant10/1 -> Add7/2
  Constant8/1 -> Add10/1
  MATLAB Function3/1(y) -> Add11/2
  MATLAB Function1/1(y) -> Add8/1, Display9/1
  Add10/1 -> Scope3/2, Compose String2/4
  String to ASCII/1 -> Signal/1
  Add8/1 -> Scope3/3, Compose String2/6
  Compose String2/1 -> String to ASCII/1
  Constant5/1 -> Add8/2
  Constant7/1 -> Add11/1
  水平扇动1/1 -> ?
  In1/1 -> Gain3/1
  R_Pit_Ang/1 -> Add10/3
  L_Pit_Ang/1 -> Add11/3
  垂直扇动1/1 -> Compose String2/5
  垂直扇动3/1 -> Compose String2/2

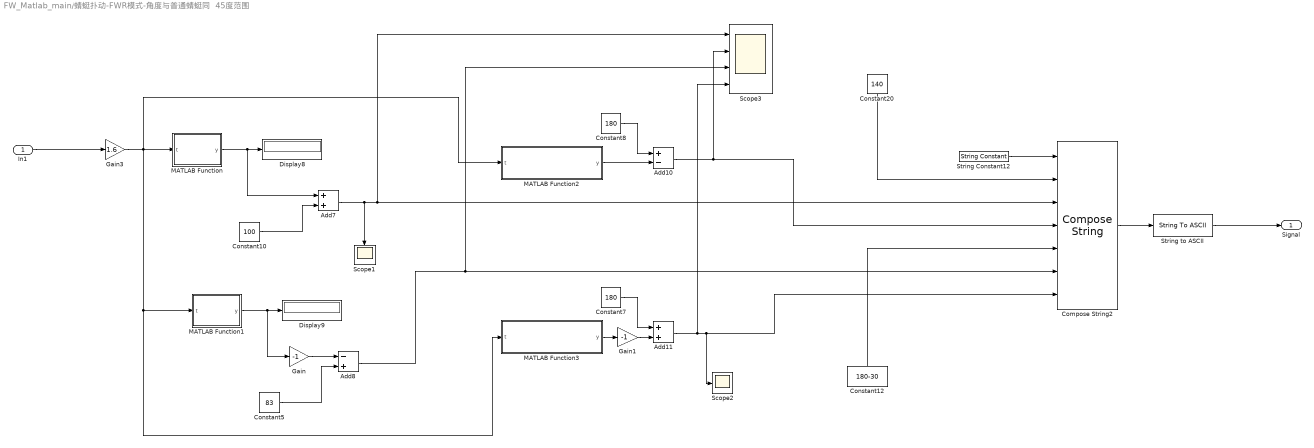
== system FW_Matlab_main/蜻蜓扑动-FWR模式-角度与普通蜻蜓同  45度范围 ==
  In1 : Inport
  Add10 : Sum  Inputs=+-
  Add11 : Sum
  Add7 : Sum
  Add8 : Sum  Inputs=-+
  Compose String2 : ComposeString  Format="\"%s%f %f %f %f %f %f\""
  Constant10 : Constant  Value=100
  Constant12 : Constant  Value=180-30
  Constant20 : Constant  Value=140
  Constant5 : Constant  Value=83
  Constant7 : Constant  Value=180
  Constant8 : Constant  Value=180
  Display8 : Display
  Display9 : Display
  Gain : Gain  Gain=-1
  Gain1 : Gain  Gain=-1
  Gain3 : Gain  Gain=1.6
  MATLAB Function : MATLAB Function  TreatAsAtomicUnit=on
  MATLAB Function1 : MATLAB Function  TreatAsAtomicUnit=on
  MATLAB Function2 : MATLAB Function  TreatAsAtomicUnit=on
  MATLAB Function3 : MATLAB Function  TreatAsAtomicUnit=on
  Scope1 : Scope
  Scope2 : Scope
  Scope3 : Scope  NumInputPorts=4
  String Constant12 : StringConstant  String="\"T\""
  String to ASCII : StringToASCII  OutputVectorSize=80
  Signal : Outport
  wires:
  Add11/1 -> Compose String2/7, Scope2/1, Scope3/4
  Gain3/1 -> MATLAB Function3/1(t), MATLAB Function1/1(t), MATLAB Function2/1(t), MATLAB Function/1(t)
  String Constant12/1 -> Compose String2/1
  Add7/1 -> Scope1/1, Compose String2/3, Scope3/1
  MATLAB Function/1(y) -> Add7/1, Display8/1
  Constant20/1 -> Compose String2/2
  MATLAB Function2/1(y) -> Add10/2
  Constant10/1 -> Add7/2
  Constant8/1 -> Add10/1
  MATLAB Function3/1(y) -> Gain1/1
  MATLAB Function1/1(y) -> Gain/1, Display9/1
  Add10/1 -> Scope3/2, Compose String2/4
  String to ASCII/1 -> Signal/1
  Add8/1 -> Scope3/3, Compose String2/6
  Compose String2/1 -> String to ASCII/1
  Constant5/1 -> Add8/2
  Constant7/1 -> Add11/1
  Constant12/1 -> Compose String2/5
  In1/1 -> Gain3/1
  Gain/1 -> Add8/1
  Gain1/1 -> Add11/2

== system FW_Matlab_main/蜻蜓扑动-VTOL模式 45度范围 ==
  In1 : Inport
  Add10 : Sum  Inputs=+-
  Add11 : Sum
  Add7 : Sum
  Add8 : Sum  Inputs=-+
  Compose String2 : ComposeString  Format="\"%s%f %f %f %f %f %f\""
  Constant10 : Constant  Value=100
  Constant12 : Constant  Value=30
  Constant20 : Constant  Value=140
  Constant5 : Constant  Value=83
  Constant7 : Constant  Value=0
  Constant8 : Constant  Value=180
  Display8 : Display
  Display9 : Display
  Gain3 : Gain  Gain=1.6
  MATLAB Function : MATLAB Function  TreatAsAtomicUnit=on
  MATLAB Function1 : MATLAB Function  TreatAsAtomicUnit=on
  MATLAB Function2 : MATLAB Function  TreatAsAtomicUnit=on
  MATLAB Function3 : MATLAB Function  TreatAsAtomicUnit=on
  Scope1 : Scope
  Scope2 : Scope
  Scope3 : Scope  NumInputPorts=4
  String Constant12 : StringConstant  String="\"T\""
  String to ASCII : StringToASCII  OutputVectorSize=80
  Signal : Outport
  wires:
  Add11/1 -> Compose String2/7, Scope2/1, Scope3/4
  Gain3/1 -> MATLAB Function3/1(t), MATLAB Function1/1(t), MATLAB Function2/1(t), MATLAB Function/1(t)
  String Constant12/1 -> Compose String2/1
  Add7/1 -> Scope1/1, Compose String2/3, Scope3/1
  MATLAB Function/1(y) -> Add7/1, Display8/1
  Constant20/1 -> Compose String2/2
  MATLAB Function2/1(y) -> Add10/2
  Constant10/1 -> Add7/2
  Constant8/1 -> Add10/1
  MATLAB Function3/1(y) -> Add11/2
  MATLAB Function1/1(y) -> Add8/1, Display9/1
  Add10/1 -> Scope3/2, Compose String2/4
  String to ASCII/1 -> Signal/1
  Add8/1 -> Scope3/3, Compose String2/6
  Compose String2/1 -> String to ASCII/1
  Constant5/1 -> Add8/2
  Constant7/1 -> Add11/1
  Constant12/1 -> Compose String2/5
  In1/1 -> Gain3/1

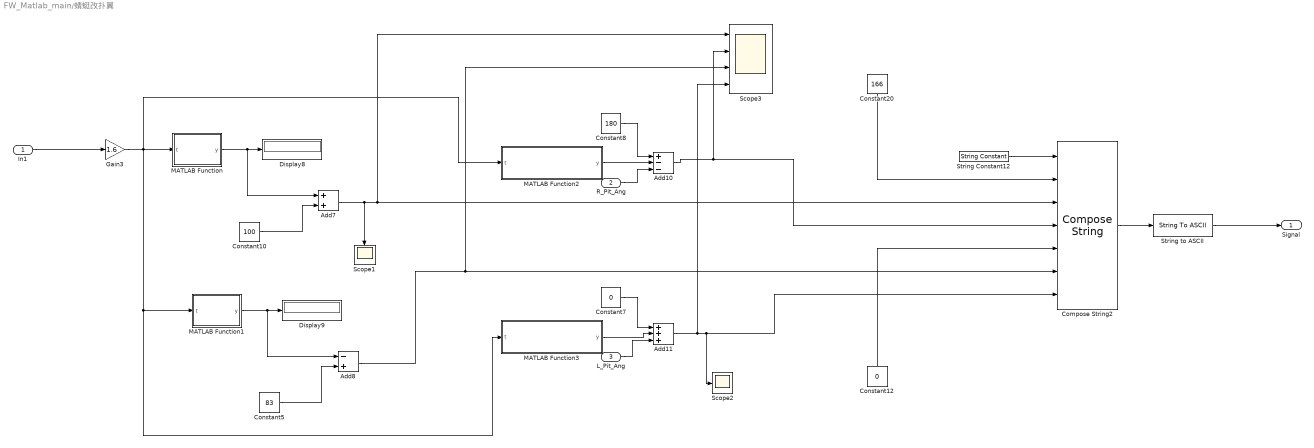
== system FW_Matlab_main/蜻蜓改扑翼 ==
  In1 : Inport
  R_Pit_Ang : Inport  Port=2
  L_Pit_Ang : Inport  Port=3
  Add10 : Sum  Inputs=+--
  Add11 : Sum  Inputs=+++
  Add7 : Sum
  Add8 : Sum  Inputs=-+
  Compose String2 : ComposeString  Format="\"%s%f %f %f %f %f %f\""
  Constant10 : Constant  Value=100
  Constant12 : Constant  Value=0
  Constant20 : Constant  Value=166
  Constant5 : Constant  Value=83
  Constant7 : Constant  Value=0
  Constant8 : Constant  Value=180
  Display8 : Display
  Display9 : Display
  Gain3 : Gain  Gain=1.6
  MATLAB Function : MATLAB Function  TreatAsAtomicUnit=on
  MATLAB Function1 : MATLAB Function  TreatAsAtomicUnit=on
  MATLAB Function2 : MATLAB Function  TreatAsAtomicUnit=on
  MATLAB Function3 : MATLAB Function  TreatAsAtomicUnit=on
  Scope1 : Scope
  Scope2 : Scope
  Scope3 : Scope  NumInputPorts=4
  String Constant12 : StringConstant  String="\"T\""
  String to ASCII : StringToASCII  OutputVectorSize=80
  Signal : Outport
  wires:
  Add11/1 -> Compose String2/7, Scope2/1, Scope3/4
  Gain3/1 -> MATLAB Function3/1(t), MATLAB Function1/1(t), MATLAB Function2/1(t), MATLAB Function/1(t)
  String Constant12/1 -> Compose String2/1
  Add7/1 -> Scope1/1, Compose String2/3, Scope3/1
  MATLAB Function/1(y) -> Add7/1, Display8/1
  Constant20/1 -> Compose String2/2
  MATLAB Function2/1(y) -> Add10/2
  Constant10/1 -> Add7/2
  Constant8/1 -> Add10/1
  MATLAB Function3/1(y) -> Add11/2
  MATLAB Function1/1(y) -> Add8/1, Display9/1
  Add10/1 -> Scope3/2, Compose String2/4
  String to ASCII/1 -> Signal/1
  Add8/1 -> Scope3/3, Compose String2/6
  Compose String2/1 -> String to ASCII/1
  Constant5/1 -> Add8/2
  Constant7/1 -> Add11/1
  Constant12/1 -> Compose String2/5
  In1/1 -> Gain3/1
  R_Pit_Ang/1 -> Add10/3
  L_Pit_Ang/1 -> Add11/3

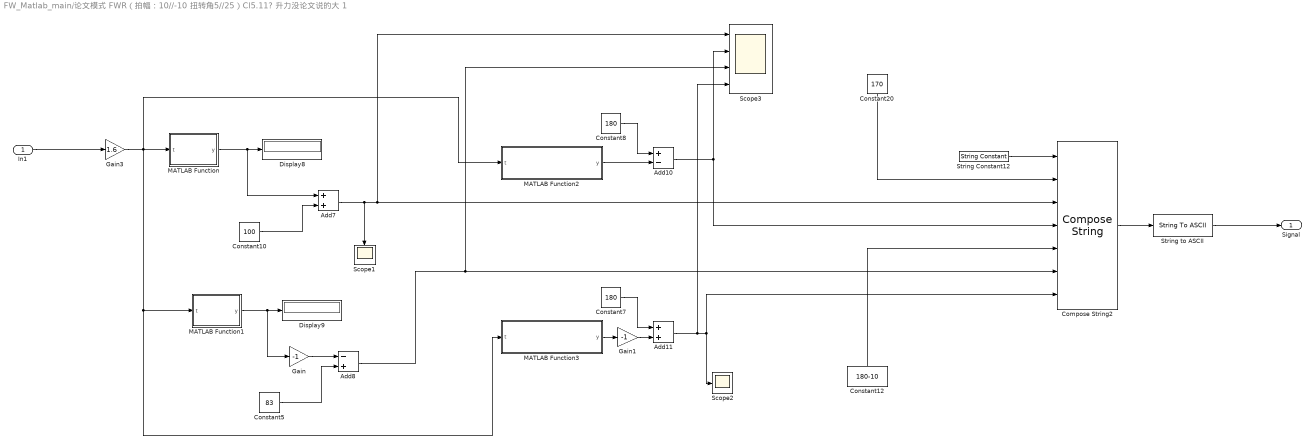
== system FW_Matlab_main/论文模式 FWR（拍幅：10//-10 扭转角5//25）Cl5.11? 升力没论文说的大 1 ==
  In1 : Inport
  Add10 : Sum  Inputs=+-
  Add11 : Sum
  Add7 : Sum
  Add8 : Sum  Inputs=-+
  Compose String2 : ComposeString  Format="\"%s%f %f %f %f %f %f\""
  Constant10 : Constant  Value=100
  Constant12 : Constant  Value=180-10
  Constant20 : Constant  Value=170
  Constant5 : Constant  Value=83
  Constant7 : Constant  Value=180
  Constant8 : Constant  Value=180
  Display8 : Display
  Display9 : Display
  Gain : Gain  Gain=-1
  Gain1 : Gain  Gain=-1
  Gain3 : Gain  Gain=1.6
  MATLAB Function : MATLAB Function  TreatAsAtomicUnit=on
  MATLAB Function1 : MATLAB Function  TreatAsAtomicUnit=on
  MATLAB Function2 : MATLAB Function  TreatAsAtomicUnit=on
  MATLAB Function3 : MATLAB Function  TreatAsAtomicUnit=on
  Scope1 : Scope
  Scope2 : Scope
  Scope3 : Scope  NumInputPorts=4
  String Constant12 : StringConstant  String="\"T\""
  String to ASCII : StringToASCII  OutputVectorSize=80
  Signal : Outport
  wires:
  Gain3/1 -> MATLAB Function3/1(t), MATLAB Function1/1(t), MATLAB Function2/1(t), MATLAB Function/1(t)
  String Constant12/1 -> Compose String2/1
  MATLAB Function/1(y) -> Add7/1, Display8/1
  Constant20/1 -> Compose String2/2
  MATLAB Function2/1(y) -> Add10/2
  Constant10/1 -> Add7/2
  Constant8/1 -> Add10/1
  MATLAB Function3/1(y) -> Gain1/1
  MATLAB Function1/1(y) -> Gain/1, Display9/1
  String to ASCII/1 -> Signal/1
  Compose String2/1 -> String to ASCII/1
  Constant5/1 -> Add8/2
  Constant7/1 -> Add11/1
  Constant12/1 -> Compose String2/5
  In1/1 -> Gain3/1
  Gain/1 -> Add8/1
  Gain1/1 -> Add11/2
  Add7/1 -> Scope1/1, Compose String2/3, Scope3/1
  Add8/1 -> Compose String2/6, Scope3/3
  Add10/1 -> Compose String2/4, Scope3/2
  Add11/1 -> Compose String2/7, Scope2/1, Scope3/4

== system FW_Matlab_main/FWR_Z_AXIS UDP/If Action Subsystem1 ==
  In1 : Inport
  Action Port : ActionPort  ActionPortLabel=if(u1 == 0)
  Out1 : Outport
  wires:
  In1/1 -> Out1/1

== system FW_Matlab_main/启动测力台 UDP  接收 /If Action Subsystem4 ==
  In1 : Inport
  Action Port : ActionPort  ActionPortLabel=case [ 0 ]:
  Out1 : Outport
  wires:
  In1/1 -> Out1/1

== matlab function FW_Matlab_main/蜻蜓扑动-VTOL模式 45度范围/MATLAB Function1 ==
  data: t input; y output
function y = back_flap(t)
y=15+30*cos((226.08*t+180)*(pi/180));
end

== matlab function FW_Matlab_main/10.27 想做对称推力测试/MATLAB Function ==
  data: t input; y output
function y = back_flap(t)
y=60*cos((226.08*t+180)*(pi/180));
end

== matlab function FW_Matlab_main/10.27 想做对称推力测试/MATLAB Function1 ==
  data: t input; y output
function y = back_flap(t)
y=60*cos((226.08*t+180)*(pi/180));
end

== matlab function FW_Matlab_main/10.27 想做对称推力测试/MATLAB Function2 ==
  data: t input; y output
function y = back_flap_twist(t)
  sita_u=90+30;   %上扑角度
  sita_d=90-30;   %下扑角度
  delta_T=0.4;
  T=1.6;
  sita_b_value=0;
  if t>=-delta_T/2 && t<=delta_T/2
    sita_b_value=(sita_u+sita_d)/2+((sita_u-sita_d)/2)*sin(3.14*t/delta_T);
  end
   if t>=delta_T/2 && t<=(T-delta_T)/2
    sita_b_value=sita_u;
   end
   if t>=(T-delta_T)/2 && t<=(T+delta_T)/2
    sita_b_value=(sita_u+sita_d)/2+((sita_u-sita_d)/2)*sin(3.14*(T/2-t)/delta_T);
   end
   if t>=(T+delta_T)/2 && t<=T-delta_T/2
    sita_b_value=sita_d;
   end
   if t>=T-delta_T/2 && t<=T
    sita_b_value=(sita_u+sita_d)/2+((sita_u-sita_d)/2)*sin(3.14*t/delta_T);
   end
   y=sita_b_value;
end

== matlab function FW_Matlab_main/10.27 想做对称推力测试/MATLAB Function3 ==
  data: t input; y output
function y = back_flap_twist(t)
  sita_u=90+30;   %上扑角度
  sita_d=90-30;   %下扑角度
  delta_T=0.4;
  T=1.6;
  sita_b_value=0;
  if t>=-delta_T/2 && t<=delta_T/2
    sita_b_value=(sita_u+sita_d)/2+((sita_u-sita_d)/2)*sin(3.14*t/delta_T);
  end
   if t>=delta_T/2 && t<=(T-delta_T)/2
    sita_b_value=sita_u;
   end
   if t>=(T-delta_T)/2 && t<=(T+delta_T)/2
    sita_b_value=(sita_u+sita_d)/2+((sita_u-sita_d)/2)*sin(3.14*(T/2-t)/delta_T);
   end
   if t>=(T+delta_T)/2 && t<=T-delta_T/2
    sita_b_value=sita_d;
   end
   if t>=T-delta_T/2 && t<=T
    sita_b_value=(sita_u+sita_d)/2+((sita_u-sita_d)/2)*sin(3.14*t/delta_T);
   end
   y=sita_b_value;
end

== matlab function FW_Matlab_main/优化中 FWR（当前最优）10.29后，改了扭转角度/MATLAB Function ==
  data: t input; y output
function y = back_flap(t)
y=30+60*cos((226.08*t+180)*(pi/180));
end

== matlab function FW_Matlab_main/优化中 FWR（当前最优）10.29后，改了扭转角度/MATLAB Function1 ==
  data: t input; y output
function y = back_flap(t)
y=30+60*cos((226.08*t+180)*(pi/180));
end

== matlab function FW_Matlab_main/优化中 FWR（当前最优）10.29后，改了扭转角度/MATLAB Function2 ==
  data: t input; y output
function y = back_flap_twist(t)
  sita_u=90+25;   %上扑角度
  sita_d=90-10;   %下扑角度
  delta_T=0.4;
  T=1.6;
  sita_b_value=0;
  if t>=-delta_T/2 && t<=delta_T/2
    sita_b_value=(sita_u+sita_d)/2+((sita_u-sita_d)/2)*sin(3.14*t/delta_T);
  end
   if t>=delta_T/2 && t<=(T-delta_T)/2
    sita_b_value=sita_u;
   end
   if t>=(T-delta_T)/2 && t<=(T+delta_T)/2
    sita_b_value=(sita_u+sita_d)/2+((sita_u-sita_d)/2)*sin(3.14*(T/2-t)/delta_T);
   end
   if t>=(T+delta_T)/2 && t<=T-delta_T/2
    sita_b_value=sita_d;
   end
   if t>=T-delta_T/2 && t<=T
    sita_b_value=(sita_u+sita_d)/2+((sita_u-sita_d)/2)*sin(3.14*t/delta_T);
   end
   y=sita_b_value;
end

== matlab function FW_Matlab_main/优化中 FWR（当前最优）10.29后，改了扭转角度/MATLAB Function3 ==
  data: t input; y output
function y = back_flap_twist(t)
  sita_u=90+25;   %上扑角度
  sita_d=90-10;   %下扑角度
  delta_T=0.4;
  T=1.6;
  sita_b_value=0;
  if t>=-delta_T/2 && t<=delta_T/2
    sita_b_value=(sita_u+sita_d)/2+((sita_u-sita_d)/2)*sin(3.14*t/delta_T);
  end
   if t>=delta_T/2 && t<=(T-delta_T)/2
    sita_b_value=sita_u;
   end
   if t>=(T-delta_T)/2 && t<=(T+delta_T)/2
    sita_b_value=(sita_u+sita_d)/2+((sita_u-sita_d)/2)*sin(3.14*(T/2-t)/delta_T);
   end
   if t>=(T+delta_T)/2 && t<=T-delta_T/2
    sita_b_value=sita_d;
   end
   if t>=T-delta_T/2 && t<=T
    sita_b_value=(sita_u+sita_d)/2+((sita_u-sita_d)/2)*sin(3.14*t/delta_T);
   end
   y=sita_b_value;
end

== matlab function FW_Matlab_main/蜻蜓改扑翼/MATLAB Function ==
  data: t input; y output
function y = back_flap(t)
y=30+60*cos((226.08*t+180)*(pi/180));
end

== matlab function FW_Matlab_main/蜻蜓改扑翼/MATLAB Function1 ==
  data: t input; y output
function y = back_flap(t)
y=30+60*cos((226.08*t+180)*(pi/180));
end

== matlab function FW_Matlab_main/蜻蜓扑动-VTOL模式 45度范围/MATLAB Function ==
  data: t input; y output
function y = back_flap(t)
y=15+30*cos((226.08*t+180)*(pi/180));
end

== matlab function FW_Matlab_main/蜻蜓改扑翼/MATLAB Function2 ==
  data: t input; y output
function y = back_flap_twist(t)
  sita_u=90+45;   %上扑角度
  sita_d=90-5;   %下扑角度
  delta_T=0.4;
  T=1.6;
  sita_b_value=0;
  if t>=-delta_T/2 && t<=delta_T/2
    sita_b_value=(sita_u+sita_d)/2+((sita_u-sita_d)/2)*sin(3.14*t/delta_T);
  end
   if t>=delta_T/2 && t<=(T-delta_T)/2
    sita_b_value=sita_u;
   end
   if t>=(T-delta_T)/2 && t<=(T+delta_T)/2
    sita_b_value=(sita_u+sita_d)/2+((sita_u-sita_d)/2)*sin(3.14*(T/2-t)/delta_T);
   end
   if t>=(T+delta_T)/2 && t<=T-delta_T/2
    sita_b_value=sita_d;
   end
   if t>=T-delta_T/2 && t<=T
    sita_b_value=(sita_u+sita_d)/2+((sita_u-sita_d)/2)*sin(3.14*t/delta_T);
   end
   y=sita_b_value;
end

== matlab function FW_Matlab_main/蜻蜓改扑翼/MATLAB Function3 ==
  data: t input; y output
function y = back_flap_twist(t)
  sita_u=90+45;   %上扑角度
  sita_d=90-5;   %下扑角度
  delta_T=0.4;
  T=1.6;
  sita_b_value=0;
  if t>=-delta_T/2 && t<=delta_T/2
    sita_b_value=(sita_u+sita_d)/2+((sita_u-sita_d)/2)*sin(3.14*t/delta_T);
  end
   if t>=delta_T/2 && t<=(T-delta_T)/2
    sita_b_value=sita_u;
   end
   if t>=(T-delta_T)/2 && t<=(T+delta_T)/2
    sita_b_value=(sita_u+sita_d)/2+((sita_u-sita_d)/2)*sin(3.14*(T/2-t)/delta_T);
   end
   if t>=(T+delta_T)/2 && t<=T-delta_T/2
    sita_b_value=sita_d;
   end
   if t>=T-delta_T/2 && t<=T
    sita_b_value=(sita_u+sita_d)/2+((sita_u-sita_d)/2)*sin(3.14*t/delta_T);
   end
   y=sita_b_value;
end

== matlab function FW_Matlab_main/优化中 FWR- 尝试姿态控制-小拍动幅度-新小幅度（周期变距）/MATLAB Function ==
  data: t input; y output
function y = back_flap(t)
y=30+30*cos((226.08*t+180)*(pi/180));
end

== matlab function FW_Matlab_main/优化中 FWR- 尝试姿态控制-小拍动幅度-新小幅度（周期变距）/MATLAB Function1 ==
  data: t input; y output
function y = back_flap(t)
y=30+30*cos((226.08*t+180)*(pi/180));
end

== matlab function FW_Matlab_main/优化中 FWR- 尝试姿态控制-小拍动幅度-新小幅度（周期变距）/MATLAB Function2 ==
  data: t input; y output
function y = back_flap_twist(t)
  sita_u=90+45;   %上扑角度
  sita_d=90-5;   %下扑角度
  delta_T=0.4;
  T=1.6;
  sita_b_value=0;
  if t>=-delta_T/2 && t<=delta_T/2
    sita_b_value=(sita_u+sita_d)/2+((sita_u-sita_d)/2)*sin(3.14*t/delta_T);
  end
   if t>=delta_T/2 && t<=(T-delta_T)/2
    sita_b_value=sita_u;
   end
   if t>=(T-delta_T)/2 && t<=(T+delta_T)/2
    sita_b_value=(sita_u+sita_d)/2+((sita_u-sita_d)/2)*sin(3.14*(T/2-t)/delta_T);
   end
   if t>=(T+delta_T)/2 && t<=T-delta_T/2
    sita_b_value=sita_d;
   end
   if t>=T-delta_T/2 && t<=T
    sita_b_value=(sita_u+sita_d)/2+((sita_u-sita_d)/2)*sin(3.14*t/delta_T);
   end
   y=sita_b_value;
end

== matlab function FW_Matlab_main/优化中 FWR- 尝试姿态控制-小拍动幅度-新小幅度（周期变距）/MATLAB Function3 ==
  data: t input; y output
function y = back_flap_twist(t)
  sita_u=90+45;   %上扑角度
  sita_d=90-5;   %下扑角度
  delta_T=0.4;
  T=1.6;
  sita_b_value=0;
  if t>=-delta_T/2 && t<=delta_T/2
    sita_b_value=(sita_u+sita_d)/2+((sita_u-sita_d)/2)*sin(3.14*t/delta_T);
  end
   if t>=delta_T/2 && t<=(T-delta_T)/2
    sita_b_value=sita_u;
   end
   if t>=(T-delta_T)/2 && t<=(T+delta_T)/2
    sita_b_value=(sita_u+sita_d)/2+((sita_u-sita_d)/2)*sin(3.14*(T/2-t)/delta_T);
   end
   if t>=(T+delta_T)/2 && t<=T-delta_T/2
    sita_b_value=sita_d;
   end
   if t>=T-delta_T/2 && t<=T
    sita_b_value=(sita_u+sita_d)/2+((sita_u-sita_d)/2)*sin(3.14*t/delta_T);
   end
   y=sita_b_value;
end

== matlab function FW_Matlab_main/Total Pitch Cyclic Control ==
  data: azimuth_ang input; blade_right output; blade_left output; Amp_Roll input; Amp_Pitch input
function [blade_right,blade_left] = T_Pit_Cyc_con(azimuth_ang,Amp_Roll,Amp_Pitch)
blade_right=Amp_Roll*sind(azimuth_ang)+Amp_Pitch*sind(azimuth_ang-90);
blade_left=Amp_Roll*sind(azimuth_ang+180)+Amp_Pitch*sind(azimuth_ang+180-90);
end

== matlab function FW_Matlab_main/优化中 FWR（当前最优）- 尝试姿态控制（周期变距）124 测王/MATLAB Function ==
  data: t input; y output
function y = back_flap(t)
y=30+60*cos((226.08*t+180)*(pi/180));
end

== matlab function FW_Matlab_main/优化中 FWR（当前最优）- 尝试姿态控制（周期变距）124 测王/MATLAB Function1 ==
  data: t input; y output
function y = back_flap(t)
y=30+60*cos((226.08*t+180)*(pi/180));
end

== matlab function FW_Matlab_main/优化中 FWR（当前最优）- 尝试姿态控制（周期变距）124 测王/MATLAB Function2 ==
  data: t input; y output
function y = back_flap_twist(t)
  sita_u=90+45;   %上扑角度
  sita_d=90-5;   %下扑角度
  delta_T=0.4;
  T=1.6;
  sita_b_value=0;
  if t>=-delta_T/2 && t<=delta_T/2
    sita_b_value=(sita_u+sita_d)/2+((sita_u-sita_d)/2)*sin(3.14*t/delta_T);
  end
   if t>=delta_T/2 && t<=(T-delta_T)/2
    sita_b_value=sita_u;
   end
   if t>=(T-delta_T)/2 && t<=(T+delta_T)/2
    sita_b_value=(sita_u+sita_d)/2+((sita_u-sita_d)/2)*sin(3.14*(T/2-t)/delta_T);
   end
   if t>=(T+delta_T)/2 && t<=T-delta_T/2
    sita_b_value=sita_d;
   end
   if t>=T-delta_T/2 && t<=T
    sita_b_value=(sita_u+sita_d)/2+((sita_u-sita_d)/2)*sin(3.14*t/delta_T);
   end
   y=sita_b_value;
end

== matlab function FW_Matlab_main/蜻蜓扑动-VTOL模式 45度范围/MATLAB Function2 ==
  data: t input; y output
function y = back_flap_twist(t)
  sita_u=170;   %上扑角度
  sita_d=65;   %下扑角度
  delta_T=0.4;
  T=1.6;
  sita_b_value=0;
  if t>=-delta_T/2 && t<=delta_T/2
    sita_b_value=(sita_u+sita_d)/2+((sita_u-sita_d)/2)*sin(3.14*t/delta_T);
  end
   if t>=delta_T/2 && t<=(T-delta_T)/2
    sita_b_value=sita_u;
   end
   if t>=(T-delta_T)/2 && t<=(T+delta_T)/2
    sita_b_value=(sita_u+sita_d)/2+((sita_u-sita_d)/2)*sin(3.14*(T/2-t)/delta_T);
   end
   if t>=(T+delta_T)/2 && t<=T-delta_T/2
    sita_b_value=sita_d;
   end
   if t>=T-delta_T/2 && t<=T
    sita_b_value=(sita_u+sita_d)/2+((sita_u-sita_d)/2)*sin(3.14*t/delta_T);
   end
   y=sita_b_value;
end

== matlab function FW_Matlab_main/优化中 FWR（当前最优）- 尝试姿态控制（周期变距）124 测王/MATLAB Function3 ==
  data: t input; y output
function y = back_flap_twist(t)
  sita_u=90+45;   %上扑角度
  sita_d=90-5;   %下扑角度
  delta_T=0.4;
  T=1.6;
  sita_b_value=0;
  if t>=-delta_T/2 && t<=delta_T/2
    sita_b_value=(sita_u+sita_d)/2+((sita_u-sita_d)/2)*sin(3.14*t/delta_T);
  end
   if t>=delta_T/2 && t<=(T-delta_T)/2
    sita_b_value=sita_u;
   end
   if t>=(T-delta_T)/2 && t<=(T+delta_T)/2
    sita_b_value=(sita_u+sita_d)/2+((sita_u-sita_d)/2)*sin(3.14*(T/2-t)/delta_T);
   end
   if t>=(T+delta_T)/2 && t<=T-delta_T/2
    sita_b_value=sita_d;
   end
   if t>=T-delta_T/2 && t<=T
    sita_b_value=(sita_u+sita_d)/2+((sita_u-sita_d)/2)*sin(3.14*t/delta_T);
   end
   y=sita_b_value;
end

== matlab function FW_Matlab_main/两翼分频控制/MATLAB Function ==
  data: t input; y output
function y = back_flap(t)
y=30+60*cos((226.08*t+180)*(pi/180));
end

== matlab function FW_Matlab_main/两翼分频控制/MATLAB Function1 ==
  data: t input; y output
function y = back_flap(t)
y=30+60*cos((226.08*t+180)*(pi/180));
end

== matlab function FW_Matlab_main/两翼分频控制/MATLAB Function2 ==
  data: t input; y output
function y = back_flap_twist(t)
  sita_u=90+45;   %上扑角度
  sita_d=90-5;   %下扑角度
  delta_T=0.4;
  T=1.6;
  sita_b_value=0;
  if t>=-delta_T/2 && t<=delta_T/2
    sita_b_value=(sita_u+sita_d)/2+((sita_u-sita_d)/2)*sin(3.14*t/delta_T);
  end
   if t>=delta_T/2 && t<=(T-delta_T)/2
    sita_b_value=sita_u;
   end
   if t>=(T-delta_T)/2 && t<=(T+delta_T)/2
    sita_b_value=(sita_u+sita_d)/2+((sita_u-sita_d)/2)*sin(3.14*(T/2-t)/delta_T);
   end
   if t>=(T+delta_T)/2 && t<=T-delta_T/2
    sita_b_value=sita_d;
   end
   if t>=T-delta_T/2 && t<=T
    sita_b_value=(sita_u+sita_d)/2+((sita_u-sita_d)/2)*sin(3.14*t/delta_T);
   end
   y=sita_b_value;
end

== matlab function FW_Matlab_main/两翼分频控制/MATLAB Function3 ==
  data: t input; y output
function y = back_flap_twist(t)
  sita_u=90+45;   %上扑角度
  sita_d=90-5;   %下扑角度
  delta_T=0.4;
  T=1.6;
  sita_b_value=0;
  if t>=-delta_T/2 && t<=delta_T/2
    sita_b_value=(sita_u+sita_d)/2+((sita_u-sita_d)/2)*sin(3.14*t/delta_T);
  end
   if t>=delta_T/2 && t<=(T-delta_T)/2
    sita_b_value=sita_u;
   end
   if t>=(T-delta_T)/2 && t<=(T+delta_T)/2
    sita_b_value=(sita_u+sita_d)/2+((sita_u-sita_d)/2)*sin(3.14*(T/2-t)/delta_T);
   end
   if t>=(T+delta_T)/2 && t<=T-delta_T/2
    sita_b_value=sita_d;
   end
   if t>=T-delta_T/2 && t<=T
    sita_b_value=(sita_u+sita_d)/2+((sita_u-sita_d)/2)*sin(3.14*t/delta_T);
   end
   y=sita_b_value;
end

== matlab function FW_Matlab_main/普通扑翼/MATLAB Function ==
  data: t input; y output
function y = back_flap(t)
%y=30+60*cos((226.08*t+180)*(pi/180));
y=60*cos((226.08*t+180)*(pi/180));
end
